simulink subsystem "WinchControl"  (R2022a)
settings: Solver=VariableStepAuto  StartTime=0.0  StopTime=10.0  RelTol=1e-3
undefined symbols (not defined in the file): constr, DE2019, DiscIntNeverNeededParam, ENVMT, params, T, winchParameter
libraries: simulink x4, slctrlblks x1
settings Model: Creator=dylaneijkelhof  LastModifiedBy=kebl6571
settings SolverCC: AlgebraicLoopSolver=TrustRegion
settings DebuggingCC: UnconnectedInputMsg=warning  UnconnectedOutputMsg=warning  UnconnectedLineMsg=warning  SFMachineParentedDataDiag=warning

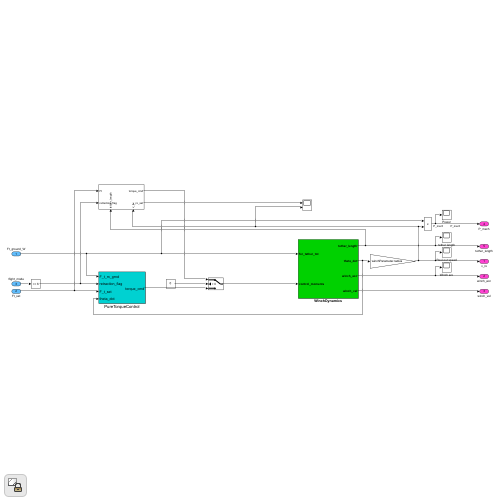
[thumbnail: Simulink's stored preview of the top-level diagram]
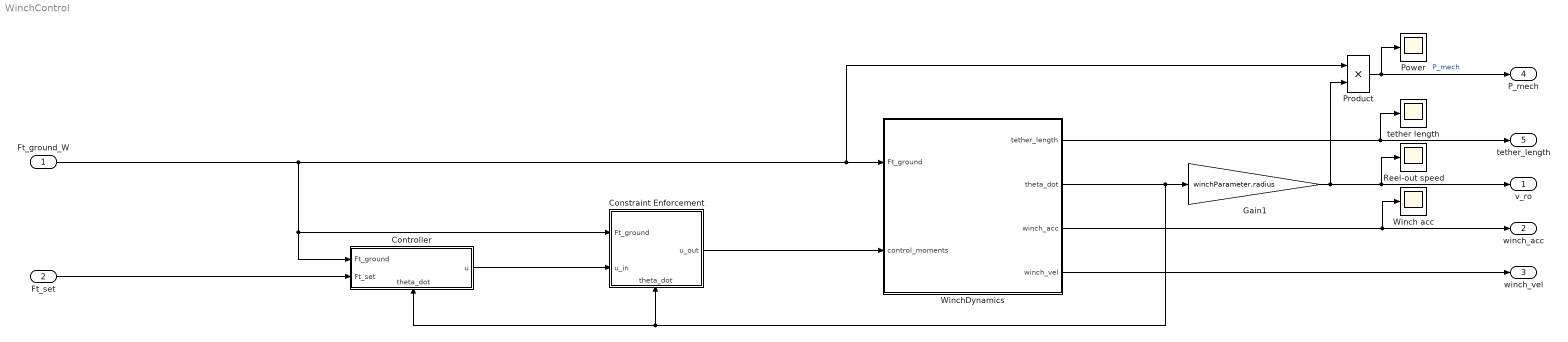
== system WinchControl ==
  Ft_ground_W : Inport  OutDataTypeStr=double  PortDimensions=1
  Ft_set : Inport  Port=2  OutDataTypeStr=double  PortDimensions=1
  Constraint Enforcement : Subsystem
      settings: PortSchema="{\"entries\":[{\"content\":{\"sides\":[{\"content\":{\"connectorIds\":[\"In1\",\"In2\"]},\"type\":\"ConnectorPlacement.EquallySpacedRectSide\",\"uuid\":\"4ca81757-379d-4af2-a12e-b37f2ca46a5b\"},{\"content\":{\"connectorIds\":[\"Out1\"],\"side\":\"RIGHT\"},\"type\":\"ConnectorPlacement.EquallySpacedRectSide\",\"uuid\":\"a27c8971-02d8-4361-b840-f786d9b80d65\"},{\"content\":{\"connectorIds\":[],\"side\":\"TOP\"},\"type\":\"ConnectorPlacement.EquallySpacedRectSide\",\"uuid\":\"4548d523-73b6-487b-9a1e-3f98b225d65f\"},{\"content\":{\"connectorIds\":[\"In3\"],\"side\":\"BOTTOM\"},\"type\":\"ConnectorPlacement.EquallySpacedRectSide\",\"uuid\":\"53183ae3-d7a4-45b9-9cb3-aa449f1749d3\"}]},\"type\":\"ConnectorPlacement.EquallySpacedConnector\",\"uuid\":\"827d45d1-147f-4a5f-a58c-ff07755b95fc\"}],\"packageUris\":[\"http://schema.mathworks.com/mf0/Connector/R2020b\"],\"version\":\"1.0\"}"
  Controller : Subsystem
      settings: PortSchema="{\"entries\":[{\"content\":{\"sides\":[{\"content\":{\"connectorIds\":[\"In1\",\"In2\"]},\"type\":\"ConnectorPlacement.EquallySpacedRectSide\",\"uuid\":\"4ca81757-379d-4af2-a12e-b37f2ca46a5b\"},{\"content\":{\"connectorIds\":[\"Out1\"],\"side\":\"RIGHT\"},\"type\":\"ConnectorPlacement.EquallySpacedRectSide\",\"uuid\":\"a27c8971-02d8-4361-b840-f786d9b80d65\"},{\"content\":{\"connectorIds\":[],\"side\":\"TOP\"},\"type\":\"ConnectorPlacement.EquallySpacedRectSide\",\"uuid\":\"4548d523-73b6-487b-9a1e-3f98b225d65f\"},{\"content\":{\"connectorIds\":[\"In3\"],\"side\":\"BOTTOM\"},\"type\":\"ConnectorPlacement.EquallySpacedRectSide\",\"uuid\":\"6d3539dc-4ef0-4ca4-abda-47de55f2d242\"}]},\"type\":\"ConnectorPlacement.EquallySpacedConnector\",\"uuid\":\"827d45d1-147f-4a5f-a58c-ff07755b95fc\"}],\"packageUris\":[\"http://schema.mathworks.com/mf0/Connector/R2020b\"],\"version\":\"1.0\"}"
  Gain1 : Gain  Gain=winchParameter.radius
  Power : Scope
  Product : Product
  Reel-out speed : Scope
  Winch acc : Scope
  WinchDynamics : Subsystem
  tether length : Scope
  v_ro : Outport  OutDataTypeStr=double  PortDimensions=1  VectorParamsAs1DForOutWhenUnconnected=off
  winch_acc : Outport  Port=2  OutDataTypeStr=double  PortDimensions=1  VectorParamsAs1DForOutWhenUnconnected=off
  winch_vel : Outport  Port=3  OutDataTypeStr=double  PortDimensions=1  VectorParamsAs1DForOutWhenUnconnected=off
  P_mech : Outport  Port=4  OutDataTypeStr=double  PortDimensions=1  VectorParamsAs1DForOutWhenUnconnected=off
  tether_length : Outport  Port=5  OutDataTypeStr=double  PortDimensions=1  VectorParamsAs1DForOutWhenUnconnected=off
  wires:
  WinchDynamics/3(winch_acc) -> winch_acc/1, Winch acc/1
  Product/1 -> P_mech/1, Power/1  "P_mech"
  WinchDynamics/4(winch_vel) -> winch_vel/1
  WinchDynamics/2(theta_dot) -> Constraint Enforcement/3(theta_dot), Controller/3(theta_dot), Gain1/1
  WinchDynamics/1(tether_length) -> tether length/1, tether_length/1
  Gain1/1 -> v_ro/1, Reel-out speed/1, Product/2
  Ft_ground_W/1 -> Constraint Enforcement/1(Ft_ground), Controller/1(Ft_ground), WinchDynamics/1(Ft_ground), Product/1
  Ft_set/1 -> Controller/2(Ft_set)
  Controller/1(u) -> Constraint Enforcement/2(u_in)
  Constraint Enforcement/1(u_out) -> WinchDynamics/2(control_moments)

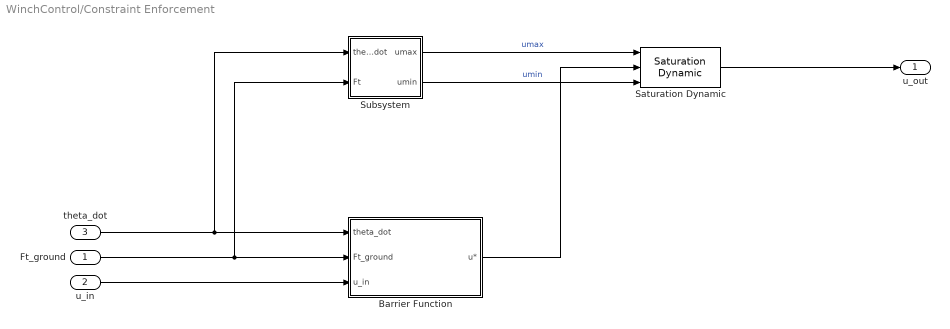
== system WinchControl/Constraint Enforcement ==
  Ft_ground : Inport
  u_in : Inport  Port=2
  theta_dot : Inport  Port=3
  Barrier Function : Subsystem
  Saturation Dynamic : simulink/Discontinuities/Saturation Dynamic  OutMin=[]  OutMax=[]  OutDataTypeStr=Inherit: Same as second input  OutDataType=fixdt(1, 16)  OutScaling=2^-10  DoSatur=off
  Subsystem : Subsystem
  u_out : Outport
  wires:
  Barrier Function/1(u*) -> Saturation Dynamic/2
  u_in/1 -> Barrier Function/3(u_in)
  Saturation Dynamic/1 -> u_out/1
  Ft_ground/1 -> Barrier Function/2(Ft_ground), Subsystem/2(Ft)
  Subsystem/2(umin) -> Saturation Dynamic/3  "umin"
  theta_dot/1 -> Barrier Function/1(theta_dot), Subsystem/1(theta_dot)
  Subsystem/1(umax) -> Saturation Dynamic/1  "umax"

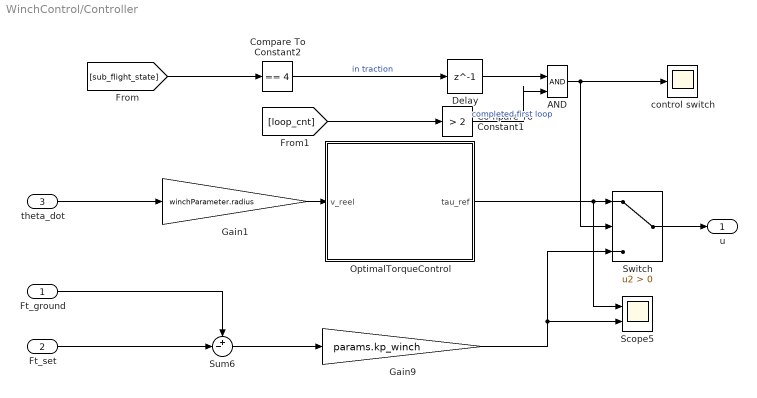
== system WinchControl/Controller ==
  Ft_ground : Inport
  Ft_set : Inport  Port=2
  theta_dot : Inport  Port=3
  AND : Logic  IconShape=distinctive  AllPortsSameDT=off  OutDataTypeStr=boolean
  Compare To Constant1 : simulink/Logic and Bit Operations/Compare To Constant  relop=>  const=2  OutDataTypeStr=boolean
  Compare To Constant2 : simulink/Logic and Bit Operations/Compare To Constant  relop===  const=4  OutDataTypeStr=boolean
  Delay : Delay  DelayLength=1
  Gain1 : Gain  Gain=winchParameter.radius
  Gain9 : Gain  Gain=params.kp_winch
  OptimalTorqueControl : MATLAB Function  TreatAsAtomicUnit=on
  Scope5 : Scope  NumInputPorts=2
  Sum6 : Sum  Inputs=+-|
  Switch : Switch  Criteria=u2 > Threshold  SaturateOnIntegerOverflow=off  InputSameDT=off
  control switch : Scope
  u : Outport
  wires:
  Gain1/1 -> OptimalTorqueControl/1(v_reel)
  Delay/1 -> AND/1
  Switch/1 -> u/1
  Compare To Constant1/1 -> AND/2  "completed first loop"
  [loop_cnt] -> Compare To Constant1/1
  AND/1 -> Switch/2, control switch/1
  Ft_ground/1 -> Sum6/1
  Ft_set/1 -> Sum6/2
  theta_dot/1 -> Gain1/1
  Sum6/1 -> Gain9/1
  [sub_flight_state] -> Compare To Constant2/1
  Gain9/1 -> Switch/3, Scope5/2
  Compare To Constant2/1 -> Delay/1  "in traction"
  OptimalTorqueControl/1(tau_ref) -> Switch/1, Scope5/1

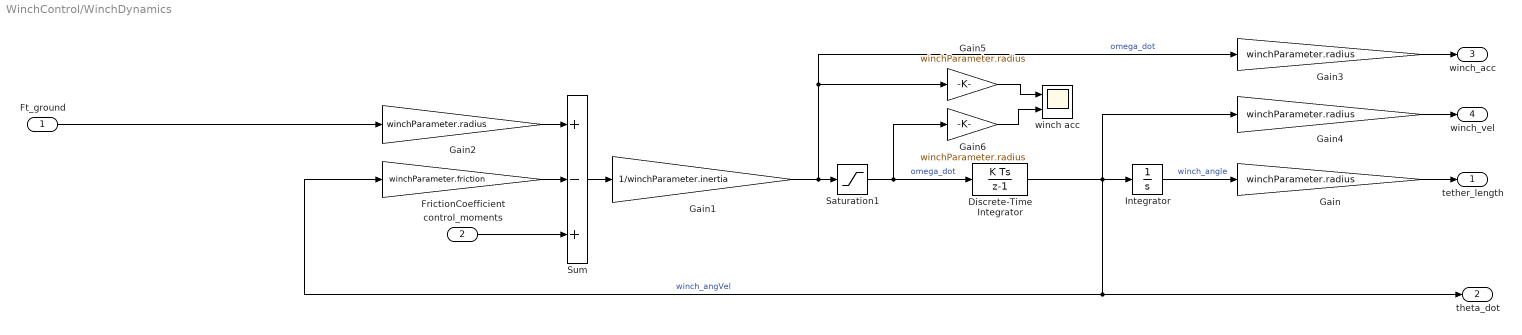
== system WinchControl/WinchDynamics ==
  Ft_ground : Inport
  control_moments : Inport  Port=2
  Discrete-Time Integrator : DiscreteIntegrator  InitialCondition=winchParameter.lj_dot_init  SampleTime=-1  LimitOutput=on  UpperSaturationLimit=constr.winchParameter.v_max/winchParameter.radius  LowerSaturationLimit=constr.winchParameter.v_min/winchParameter.radius  ICPrevOutput=DiscIntNeverNeededParam  ICPrevScaledInput=DiscIntNeverNeededParam
  FrictionCoefficient : Gain  Gain=winchParameter.friction
  Gain{,2..6} (6 alike) : Gain  Gain=winchParameter.radius
  Gain1 : Gain  Gain=1/winchParameter.inertia
  Integrator : Integrator  InitialCondition=winchParameter.winch_angle_init
  Saturation1 : Saturate  UpperLimit=constr.winchParameter.a_max/winchParameter.radius  LowerLimit=constr.winchParameter.a_min/winchParameter.radius
  Sum : Sum  Inputs=+-+
  winch acc : Scope  NumInputPorts=2
  tether_length : Outport  VectorParamsAs1DForOutWhenUnconnected=off
  theta_dot : Outport  Port=2  VectorParamsAs1DForOutWhenUnconnected=off
  winch_acc : Outport  Port=3  VectorParamsAs1DForOutWhenUnconnected=off
  winch_vel : Outport  Port=4  VectorParamsAs1DForOutWhenUnconnected=off
  wires:
  control_moments/1 -> Sum/3
  Saturation1/1 -> Gain6/1, Discrete-Time Integrator/1  "omega_dot"
  Ft_ground/1 -> Gain2/1
  Gain6/1 -> winch acc/2
  Gain5/1 -> winch acc/1
  Gain3/1 -> winch_acc/1
  Gain4/1 -> winch_vel/1
  Gain1/1 -> Gain3/1, Gain5/1, Saturation1/1  "omega_dot"
  FrictionCoefficient/1 -> Sum/2
  Discrete-Time Integrator/1 -> Integrator/1, Gain4/1, theta_dot/1, FrictionCoefficient/1  "winch_angVel"
  Integrator/1 -> Gain/1  "winch_angle"
  Sum/1 -> Gain1/1
  Gain2/1 -> Sum/1
  Gain/1 -> tether_length/1

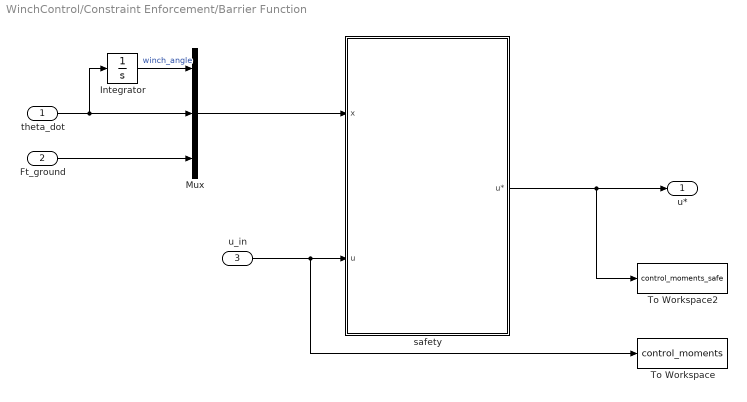
== system WinchControl/Constraint Enforcement/Barrier Function ==
  theta_dot : Inport
  Ft_ground : Inport  Port=2
  u_in : Inport  Port=3
  Integrator : Integrator  InitialCondition=winchParameter.winch_angle_init
  Mux : Mux  Inputs=3
  To Workspace : ToWorkspace  VariableName=control_moments  SaveFormat=Timeseries  SampleTime=-1
  To Workspace2 : ToWorkspace  VariableName=control_moments_safe  SaveFormat=Timeseries  SampleTime=-1
  safety : Subsystem
  u* : Outport
  wires:
  Integrator/1 -> Mux/1  "winch_angle"
  theta_dot/1 -> Mux/2, Integrator/1
  u_in/1 -> safety/2(u), To Workspace/1
  safety/1(u*) -> To Workspace2/1, u*/1
  Mux/1 -> safety/1(x)
  Ft_ground/1 -> Mux/3

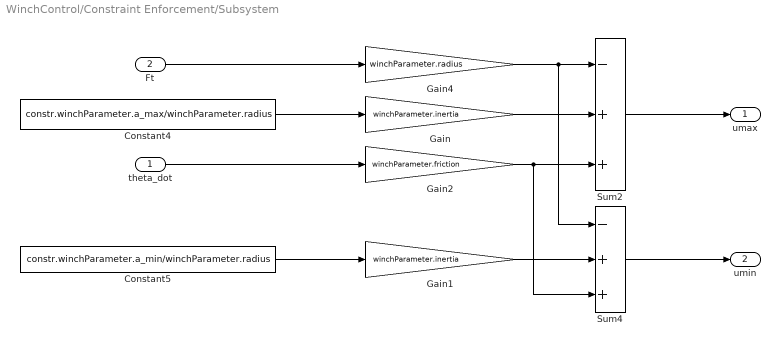
== system WinchControl/Constraint Enforcement/Subsystem ==
  theta_dot : Inport
  Ft : Inport  Port=2
  Constant4 : Constant  Value=constr.winchParameter.a_max/winchParameter.radius
  Constant5 : Constant  Value=constr.winchParameter.a_min/winchParameter.radius
  Gain : Gain  Gain=winchParameter.inertia
  Gain1 : Gain  Gain=winchParameter.inertia
  Gain2 : Gain  Gain=winchParameter.friction
  Gain4 : Gain  Gain=winchParameter.radius
  Sum2 : Sum  Inputs=-++
  Sum4 : Sum  Inputs=-++
  umax : Outport
  umin : Outport  Port=2
  wires:
  theta_dot/1 -> Gain2/1
  Gain4/1 -> Sum4/1, Sum2/1
  Ft/1 -> Gain4/1
  Sum2/1 -> umax/1
  Gain1/1 -> Sum4/2
  Gain/1 -> Sum2/2
  Constant5/1 -> Gain1/1
  Constant4/1 -> Gain/1
  Sum4/1 -> umin/1
  Gain2/1 -> Sum2/3, Sum4/3

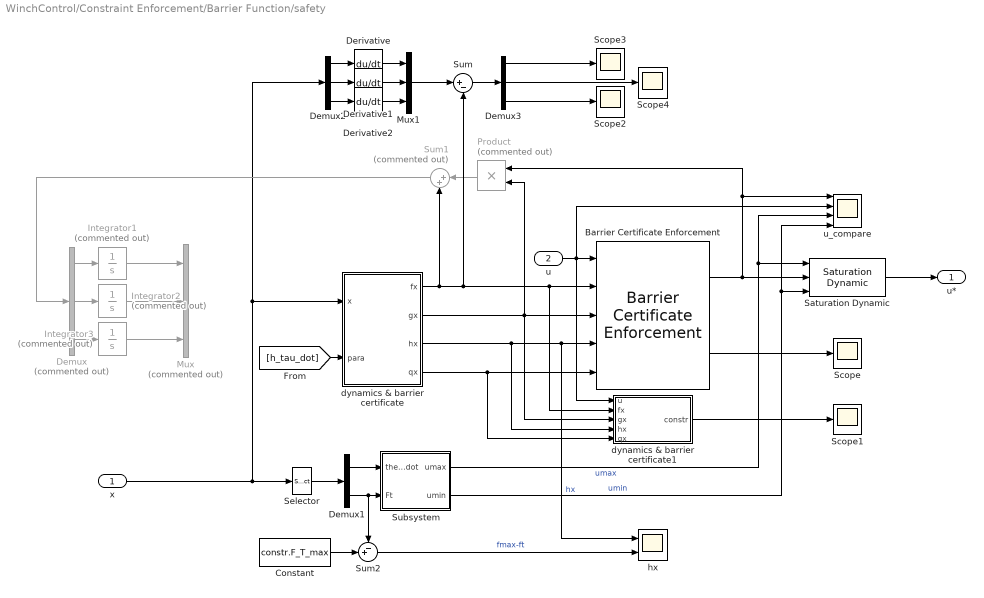
== system WinchControl/Constraint Enforcement/Barrier Function/safety ==
  x : Inport
  u : Inport  Port=2
  Barrier Certificate Enforcement : slctrlblks/Barrier Certificate Enforcement  nx=3  nu=1  nc=1  gamma=2  beta=1  external_umax=off  external_umin=off  Ts=0.001  maxiter=100  tol=1e-2  output_exitflag=on
      settings: SourceProductBaseCode=SD
  Constant : Constant  Value=constr.F_T_max
  Demux : Demux  Commented=on  Outputs=3
  Demux1 : Demux  Outputs=2
  Demux2 : Demux  Outputs=3
  Demux3 : Demux  Outputs=3
  Derivative : Derivative
  Derivative1 : Derivative
  Derivative2 : Derivative
  Integrator1 : Integrator  Commented=on  InitialCondition=winchParameter.winch_angle_init
  Integrator2 : Integrator  Commented=on  InitialCondition=winchParameter.lj_dot_init
  Integrator3 : Integrator  Commented=on
  Mux : Mux  Commented=on  Inputs=3
  Mux1 : Mux  Inputs=3
  Product : Product  Commented=on
  Saturation Dynamic : simulink/Discontinuities/Saturation Dynamic  OutMin=[]  OutMax=[]  OutDataTypeStr=Inherit: Same as second input  OutDataType=fixdt(1, 16)  OutScaling=2^-10  DoSatur=off
  Scope{,1..4} (5 alike) : Scope
  Selector : Selector  InputPortWidth=3  IndexOptions=Index vector (dialog)  Indices=[2 3]  OutputSizes=1
  Subsystem : Subsystem
  Sum : Sum  Inputs=|+-
  Sum1 : Sum  Commented=on  Inputs=|++
  Sum2 : Sum  Inputs=-+|
  dynamics & barrier certificate : MATLAB Function  TreatAsAtomicUnit=on
  dynamics & barrier certificate1 : MATLAB Function  TreatAsAtomicUnit=on
  hx : Scope  NumInputPorts=2
  u_compare : Scope  NumInputPorts=4
  u* : Outport
  wires:
  Demux3/2 -> Scope4/1
  Demux3/1 -> Scope3/1
  Demux3/3 -> Scope2/1
  Sum/1 -> Demux3/1
  Mux1/1 -> Sum/1
  Derivative/1 -> Mux1/1
  Derivative1/1 -> Mux1/2
  Derivative2/1 -> Mux1/3
  Demux2/3 -> Derivative2/1
  Demux2/2 -> Derivative1/1
  Demux2/1 -> Derivative/1
  dynamics & barrier certificate1/1(constr) -> Scope1/1
  dynamics & barrier certificate/4(qx) -> Barrier Certificate Enforcement/5, dynamics & barrier certificate1/5(qx)
  Saturation Dynamic/1 -> u*/1
  Barrier Certificate Enforcement/2 -> Scope/1
  Demux1/2 -> Subsystem/2(Ft), Sum2/1
  Demux1/1 -> Subsystem/1(theta_dot)
  Sum2/1 -> hx/2  "fmax-ft"
  Constant/1 -> Sum2/2
  Selector/1 -> Demux1/1
  x/1 -> Selector/1, dynamics & barrier certificate/1(x), Demux2/1
  Barrier Certificate Enforcement/1 -> Saturation Dynamic/2, Product/1, u_compare/1
  dynamics & barrier certificate/2(gx) -> Barrier Certificate Enforcement/3, Product/2, dynamics & barrier certificate1/3(gx)
  Product/1 -> Sum1/1
  u/1 -> u_compare/2, Barrier Certificate Enforcement/1, dynamics & barrier certificate1/1(u)
  dynamics & barrier certificate/3(hx) -> Barrier Certificate Enforcement/4, hx/1, dynamics & barrier certificate1/4(hx)  "hx"
  Subsystem/1(umax) -> u_compare/3, Saturation Dynamic/1  "umax"
  Subsystem/2(umin) -> Saturation Dynamic/3, u_compare/4  "umin"
  Integrator1/1 -> Mux/1
  [h_tau_dot] -> dynamics & barrier certificate/2(para)
  Sum1/1 -> Demux/1
  Demux/1 -> Integrator1/1
  Integrator2/1 -> Mux/2
  Demux/3 -> Integrator3/1
  Integrator3/1 -> Mux/3
  Demux/2 -> Integrator2/1
  dynamics & barrier certificate/1(fx) -> Barrier Certificate Enforcement/2, dynamics & barrier certificate1/2(fx), Sum/2, Sum1/2

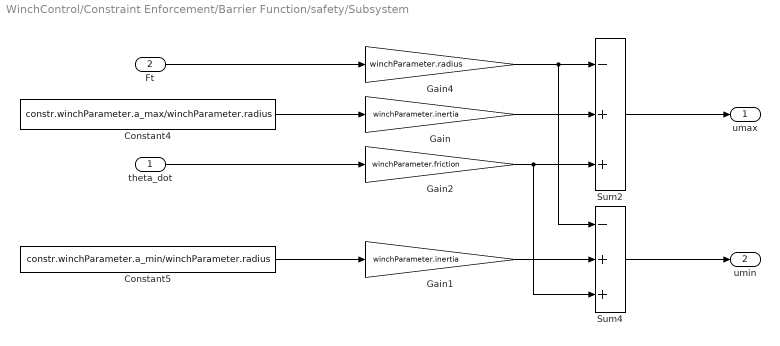
== system WinchControl/Constraint Enforcement/Barrier Function/safety/Subsystem ==
  theta_dot : Inport
  Ft : Inport  Port=2
  Constant4 : Constant  Value=constr.winchParameter.a_max/winchParameter.radius
  Constant5 : Constant  Value=constr.winchParameter.a_min/winchParameter.radius
  Gain : Gain  Gain=winchParameter.inertia
  Gain1 : Gain  Gain=winchParameter.inertia
  Gain2 : Gain  Gain=winchParameter.friction
  Gain4 : Gain  Gain=winchParameter.radius
  Sum2 : Sum  Inputs=-++
  Sum4 : Sum  Inputs=-++
  umax : Outport
  umin : Outport  Port=2
  wires:
  theta_dot/1 -> Gain2/1
  Gain4/1 -> Sum4/1, Sum2/1
  Ft/1 -> Gain4/1
  Sum2/1 -> umax/1
  Gain1/1 -> Sum4/2
  Gain/1 -> Sum2/2
  Constant5/1 -> Gain1/1
  Constant4/1 -> Gain/1
  Sum4/1 -> umin/1
  Gain2/1 -> Sum2/3, Sum4/3

== matlab function WinchControl/Constraint Enforcement/Barrier Function/safety/dynamics & barrier certificate ==
  data: x input; fx output; para input; gx output; T parameter; winchParameter parameter; hx output; qx output; constr parameter
function [fx, gx, hx, qx] = fcn(x, para, T, winchParameter, constr)
% simplified dynamcis of the winch
theta = x(1);
omega = x(2);
Ft    = x(3); % force at ground (approximated to be same as force at kite)

nu = winchParameter.friction;
Jw = winchParameter.inertia;
rw = winchParameter.radius;
ls = rw*theta; % tether length

h_tau_dot = para(1);

gx = zeros(3,1);
gx(2) = 1/Jw;
fx = zeros(3,1);

fx(1) = omega;
fx(2) = rw/Jw * Ft - nu/Jw * omega;
fx(3) = T.A * T.E/ls *(h_tau_dot - rw * omega) - rw/ls *Ft*omega;
% Ft_dot_dot = -omega/theta^2 *(T.A * T.E *(h_tau_dot/rw - omega) - Ft*omega)...
%               -1/theta*((T.A * T.E + Ft) *fx(2) + fx(3)*omega);

h_tau_dot_worst = 15;
fx_3_worst = T.A * T.E/ls *(h_tau_dot_worst - rw * omega) - rw/ls *Ft*omega;

horizon = 1; % time horizon
Ft_margin = 0.03 * constr.F_T_max; % 2% of the max tether force
if fx_3_worst > 0 % If the force is increasing
    hx = constr.F_T_max - Ft_margin - Ft - fx(3)*horizon; % First order approximation
    qx = [0,0,-1] + horizon*[1/theta^2*(T.A * T.E *(h_tau_dot_worst/rw - omega) - Ft*omega),...
                             1/theta*(T.A * T.E + Ft),...
                             1*omega/theta];
    % Assume that qx part with Ft_dot_dot is negligable.
else
    hx = constr.F_T_max - Ft_margin - Ft;
    qx = [0,0,-1]; 
end

== matlab function WinchControl/Constraint Enforcement/Barrier Function/safety/dynamics & barrier certificate1 ==
  data: u input; constr output; fx input; gx input; hx input; qx input
function constr = fcn(u, fx, gx, hx, qx)
% output the barrier constraint

gamma = 2;
beta = 1;

constr = qx*fx + qx*gx*u+gamma *hx^beta;

== matlab function WinchControl/Controller/OptimalTorqueControl ==
  data: v_reel input; tau_ref output; ENVMT parameter; DE2019 parameter; constr parameter; winchParameter parameter
function tau_ref = fcn(v_reel, ENVMT, DE2019, constr, winchParameter)

% From todeschiniControlRigidWing2021
% k_gen based on ideal conditions (max CL) and not current conditions, is
% that correct? This assumes that the kite is performing optimally.
% TODO: Do this more precisely.
CL_eq = constr.max_CL;
CD_eq = 0.16;  % Educated guess so that L/D is 15;
E = CL_eq / CD_eq;
k_gen = 2 * ENVMT.rhos * DE2019.S_wing * CL_eq * winchParameter.radius * E^2 * (1+1/E^2)^(3/2);

% MegAWES convention is different so we add a minus sign.
tau_ref = -k_gen * v_reel^2;
